simulink model "TotalControllerSimOld"  (R2015b)
settings: Solver=VariableStepAuto  StartTime=0.0  StopTime=t  RelTol=1e-3
values from neighbouring files (symbols this model uses):
  A12 = A(1:3,4:6)    [StateSpace.m]
  Fg = 9.81 * m    (= 9.77076)    [Parameters.m]
  Jx_changed = Jx*5    (= 0.0535)    [Parameters.m]
  Jy_changed = Jy*3    (= 0.0321)    [Parameters.m]
  Jz_changed = Jz*2    (= 0.0427)    [Parameters.m]
  kd = 9.39741e-7    (= 9.39741e-07)    [Parameters.m]
  kth = 1.32922e-5    (= 1.32922e-05)    [Parameters.m]
  L = 0.225    [Parameters.m]
  Lobs = (-place(A22',A12',[-11 -12 -13]))'    [StateSpace.m]
  m = 0.996    [Parameters.m]
  motor_tau = ts/3    (= 0.000333333333333)    [TotalController.m]
  pitch_init = 0    [plotPaper.m]    (also in plotPoster.m; plotStateSpace.m = 0.2; plotTrans.m)
  pitch_ref_time = 0    [plotPaper.m]    (also in plotPoster.m; plotStateSpace.m; plotTrans.m)
  pitch_step = 0    [plotPaper.m]    (also in plotPoster.m; plotStateSpace.m; plotTrans.m)
  roll_init = 0    [plotPaper.m]    (also in plotPoster.m; plotStateSpace.m = -0.3; plotTrans.m)
  roll_ref_time = 0    [plotPaper.m]    (also in plotPoster.m; plotStateSpace.m; plotTrans.m)
  roll_step = 0.2    [plotPaper.m]    (also in plotPoster.m = 0; plotStateSpace.m = 0; plotTrans.m = 0)
  w1_bar = sqrt(Fg/kth/4)    [Parameters.m]
  w2_bar = sqrt(Fg/kth/4)    [Parameters.m]
  w3_bar = sqrt(Fg/kth/4)    [Parameters.m]
  w4_bar = sqrt(Fg/kth/4)    [Parameters.m]
  w_max = 230    [TotalController.m]
  w_min = -161    [TotalController.m]
  x_ref_step = 1    [plotPaper.m]    (also in plotPoster.m = 0; plotStateSpace.m = 0; plotTrans.m)
  x_ref_time = 0    [plotPaper.m]    (also in plotPoster.m; plotStateSpace.m; plotTrans.m)
  xdot_ref_step = 0    [plotPaper.m]    (also in plotPoster.m; plotStateSpace.m; plotTrans.m)
  xdot_ref_time = 0    [plotPaper.m]    (also in plotPoster.m; plotStateSpace.m; plotTrans.m)
  y_ref_step = 1    [plotPaper.m]    (also in plotPoster.m = 0; plotStateSpace.m = 0; plotTrans.m = 0)
  y_ref_time = 8    [plotPaper.m]    (also in plotPoster.m = 0; plotStateSpace.m = 0; plotTrans.m = 2.5)
  yaw_init = 0    [plotPaper.m]    (also in plotPoster.m; plotStateSpace.m = -0.2; plotTrans.m)
  ydot_ref_step = 0    [plotPaper.m]    (also in plotPoster.m; plotStateSpace.m; plotTrans.m)
  ydot_ref_time = 0    [plotPaper.m]    (also in plotPoster.m; plotStateSpace.m; plotTrans.m)
  z_ref_step = 1    [plotPaper.m]    (also in plotPoster.m; plotStateSpace.m = 0; plotTrans.m)
  z_ref_time = 16    [plotPaper.m]    (also in plotPoster.m = 0; plotStateSpace.m = 0; plotTrans.m = 0)
  zdot_ref_step = 0    [plotPaper.m]    (also in plotPoster.m; plotStateSpace.m; plotTrans.m)
  zdot_ref_time = 0    [plotPaper.m]    (also in plotPoster.m; plotStateSpace.m; plotTrans.m)
undefined symbols (not defined in the file or in its folder): ZigBee
libraries: truetime x21, cstblocks x6, simulink x3
settings Model: Creator=USUARIO  LastModifiedBy=USUARIO

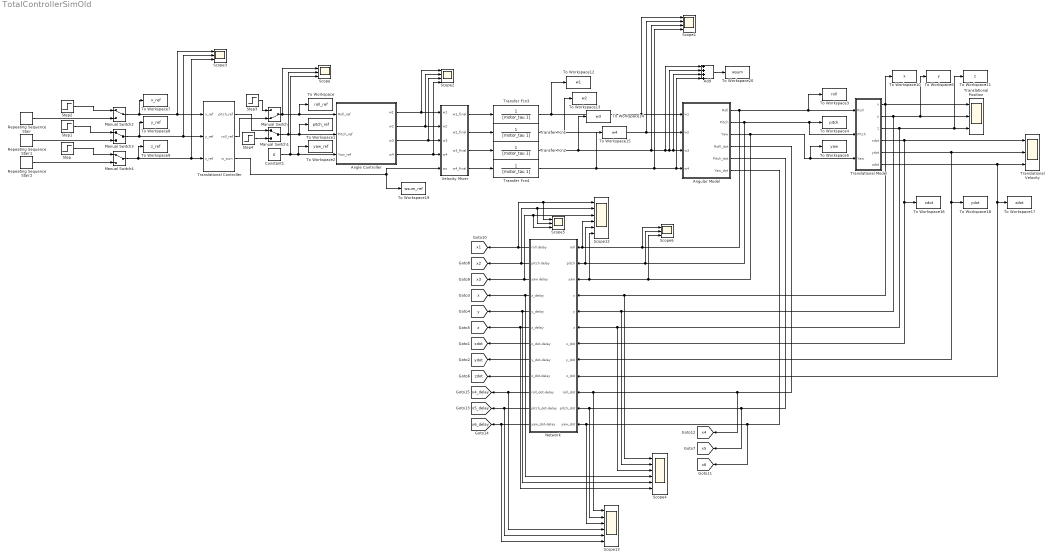
== system TotalControllerSimOld ==
  Add : Sum  Inputs=++++
  Angle Controller : Subsystem
  Angular Model : Subsystem
  Constant1 : Constant  Value=0
  Manual Switch : ManualSwitch  CurrentSetting=0
  Manual Switch{1..4} (4 alike) : ManualSwitch
  Network : Subsystem
  Repeating Sequence Stair : simulink/Sources/Repeating Sequence Stair  OutValues=input_x  tsamp=Tstep  OutMin=[]  OutMax=[]  OutDataTypeStr=double  OutputDataTypeScalingMode=double  OutDataType=fixdt(0,8)  ConRadixGroup=Best Precision: Vector-wise  OutScaling=2^-12
  Repeating Sequence Stair1 : simulink/Sources/Repeating Sequence Stair  OutValues=input_y  tsamp=Tstep  OutMin=[]  OutMax=[]  OutDataTypeStr=double  OutputDataTypeScalingMode=double  OutDataType=fixdt(0,8)  ConRadixGroup=Best Precision: Vector-wise  OutScaling=2^-12
  Repeating Sequence Stair2 : simulink/Sources/Repeating Sequence Stair  OutValues=input_z  tsamp=Tstep  OutMin=[]  OutMax=[]  OutDataTypeStr=double  OutputDataTypeScalingMode=double  OutDataType=fixdt(0,8)  ConRadixGroup=Best Precision: Vector-wise  OutScaling=2^-12
  Scope{,3,5..6} (4 alike) : Scope  NumInputPorts=3
  Scope1 : Scope  NumInputPorts=4
  Scope12 : Scope  NumInputPorts=6
  Scope13 : Scope  NumInputPorts=6
  Scope2 : Scope  NumInputPorts=4
  Scope4 : Scope  NumInputPorts=6
  Step : Step  Time=z_ref_time  After=z_ref_step  SampleTime=0
  Step1 : Step  Time=y_ref_time  After=y_ref_step  SampleTime=0
  Step2 : Step  Time=x_ref_time  After=x_ref_step  SampleTime=0
  Step3 : Step  Time=roll_ref_time  After=roll_step  SampleTime=0
  Step4 : Step  Time=pitch_ref_time  After=pitch_step  SampleTime=0
  To Workspace : ToWorkspace  VariableName=roll_ref  SaveFormat=Timeseries  SampleTime=-1
  To Workspace1 : ToWorkspace  VariableName=pitch_ref  SaveFormat=Timeseries  SampleTime=-1
  To Workspace10 : ToWorkspace  VariableName=x  SaveFormat=Timeseries  SampleTime=-1
  To Workspace11 : ToWorkspace  VariableName=z  SaveFormat=Timeseries  SampleTime=-1
  To Workspace12 : ToWorkspace  VariableName=w1  SaveFormat=Timeseries  SampleTime=-1
  To Workspace13 : ToWorkspace  VariableName=w2  SaveFormat=Timeseries  SampleTime=-1
  To Workspace14 : ToWorkspace  VariableName=w3  SaveFormat=Timeseries  SampleTime=-1
  To Workspace15 : ToWorkspace  VariableName=w4  SaveFormat=Timeseries  SampleTime=-1
  To Workspace16 : ToWorkspace  VariableName=xdot  SaveFormat=Timeseries  SampleTime=-1
  To Workspace17 : ToWorkspace  VariableName=zdot  SaveFormat=Timeseries  SampleTime=-1
  To Workspace18 : ToWorkspace  VariableName=ydot  SaveFormat=Timeseries  SampleTime=-1
  To Workspace19 : ToWorkspace  VariableName=wsum_ref  SaveFormat=Timeseries  SampleTime=-1
  To Workspace2 : ToWorkspace  VariableName=yaw_ref  SaveFormat=Timeseries  SampleTime=-1
  To Workspace20 : ToWorkspace  VariableName=wsum  SaveFormat=Timeseries  SampleTime=-1
  To Workspace3 : ToWorkspace  VariableName=roll  SaveFormat=Timeseries  SampleTime=-1
  To Workspace4 : ToWorkspace  VariableName=pitch  SaveFormat=Timeseries  SampleTime=-1
  To Workspace5 : ToWorkspace  VariableName=yaw  SaveFormat=Timeseries  SampleTime=-1
  To Workspace6 : ToWorkspace  VariableName=y  SaveFormat=Timeseries  SampleTime=-1
  To Workspace7 : ToWorkspace  VariableName=x_ref  SaveFormat=Timeseries  SampleTime=0.035
  To Workspace8 : ToWorkspace  VariableName=y_ref  SaveFormat=Timeseries  SampleTime=0.035
  To Workspace9 : ToWorkspace  VariableName=z_ref  SaveFormat=Timeseries  SampleTime=0.035
  Transfer Fcn{1..4} (4 alike) : TransferFcn  Denominator=[motor_tau 1]
  Translational Controller : Subsystem
  Translational Position : Scope  NumInputPorts=3
  Translational Velocity : Scope  NumInputPorts=3
  Translational Model : Subsystem
  Velocity Mixer : Subsystem
  tag scope: x1=global, x2=global, x3=global, x4=global, x4_delay=global, x5=global, x5_delay=global, x6=global, x6_delay=global, x=global, xdot=global, y=global, ydot=global, z=global, zdot=global
  wires:
  Constant1/1 -> Scope/3, To Workspace2/1, Angle Controller/3(Yaw_ref)
  Velocity Mixer/1(w1_final) -> Transfer Fcn3/1
  Velocity Mixer/2(w2_final) -> Transfer Fcn1/1
  Velocity Mixer/3(w3_final) -> Transfer Fcn2/1
  Velocity Mixer/4(w4_final) -> Transfer Fcn4/1
  Angle Controller/1(w1) -> Velocity Mixer/1(w1), Scope2/1
  Angle Controller/2(w2) -> Velocity Mixer/2(w2), Scope2/2
  Angle Controller/3(w3) -> Scope2/3, Velocity Mixer/3(w3)
  Angle Controller/4(w4) -> Velocity Mixer/4(w4), Scope2/4
  Angular Model/1(Roll) -> Scope12/4, Network/1(roll), Scope6/1, Translational Model/1(Roll), To Workspace3/1
  Angular Model/2(Pitch) -> Scope12/5, Network/2(pitch), Scope6/2, Translational Model/2(Pitch), To Workspace4/1
  Translational Model/1(x) -> Translational Position/1, Network/4(x), Scope4/1, To Workspace10/1
  Translational Model/2(y) -> Translational Position/2, To Workspace6/1, Network/5(y), Scope4/2
  Translational Model/3(z) -> To Workspace11/1, Translational Position/3, Network/6(z), Scope4/3
  Translational Model/4(xdot) -> Network/7(x_dot), To Workspace16/1, Translational Velocity/1
  Translational Model/5(ydot) -> Network/8(y_dot), To Workspace18/1, Translational Velocity/2
  Manual Switch1/1 -> Scope/2, To Workspace1/1, Angle Controller/2(Pitch_ref)
  Network/2(pitch delay) -> Scope5/2, Scope12/2, [x2]
  Network/1(roll delay) -> Scope5/1, Scope12/1, [x1]
  Network/3(yaw delay) -> Scope5/3, Scope12/3, [x3]
  Network/4(x_delay) -> Scope4/4, [x]
  Network/5(y_delay) -> [y], Scope4/5
  Network/6(z_delay) -> [z], Scope4/6
  Network/7(x_dot-delay) -> [xdot]
  Network/8(y_dot-delay) -> [ydot]
  Network/9(z_dot-delay) -> [zdot]
  Angular Model/3(Yaw) -> Scope12/6, Network/3(yaw), Scope6/3, Translational Model/3("Yaw "), To Workspace5/1
  Translational Model/6(zdot) -> Network/9(z_dot), To Workspace17/1, Translational Velocity/3
  Angular Model/4(Rolll_dot) -> Network/10(roll_dot), Scope13/1, [x4]
  Angular Model/6(Yaw_dot) -> [x6], Network/12(yaw_dot), Scope13/3
  Network/10(roll_dot-delay) -> Scope13/4, [x4_delay]
  Network/11(pitch_dot-delay) -> Scope13/5, [x5_delay]
  Network/12(yaw_dot-delay) -> [x6_delay], Scope13/6
  Angular Model/5(Pitch_dot) -> [x5], Network/11(pitch_dot), Scope13/2
  Manual Switch2/1 -> To Workspace7/1, Scope3/1, Translational Controller/1(x_ref)
  Manual Switch4/1 -> To Workspace9/1, Scope3/3, Translational Controller/3(z_ref)
  Manual Switch3/1 -> To Workspace8/1, Scope3/2, Translational Controller/2(y_ref)
  Translational Controller/3(w_sum) -> Velocity Mixer/5(wz), To Workspace19/1
  Step3/1 -> Manual Switch/1
  Step4/1 -> Manual Switch1/2
  Translational Controller/2(roll_ref) -> Manual Switch/2
  Translational Controller/1(pitch_ref) -> Manual Switch1/1
  Transfer Fcn3/1 -> To Workspace12/1, Scope1/1, Angular Model/1(w1)
  Transfer Fcn1/1 -> To Workspace13/1, Scope1/2, Angular Model/2(w2)
  Transfer Fcn4/1 -> To Workspace15/1, Scope1/4, Add/4, Angular Model/4(w4)
  Repeating Sequence Stair/1 -> Manual Switch2/2
  Repeating Sequence Stair1/1 -> Manual Switch3/2
  Repeating Sequence Stair2/1 -> Manual Switch4/2
  Step/1 -> Manual Switch4/1
  Step1/1 -> Manual Switch3/1
  Step2/1 -> Manual Switch2/1
  Manual Switch/1 -> Scope/1, To Workspace/1, Angle Controller/1(Roll_ref)
  Transfer Fcn2/1 -> Scope1/3, Add/1, Add/2, Add/3, Angular Model/3(w3), To Workspace14/1
  Add/1 -> To Workspace20/1

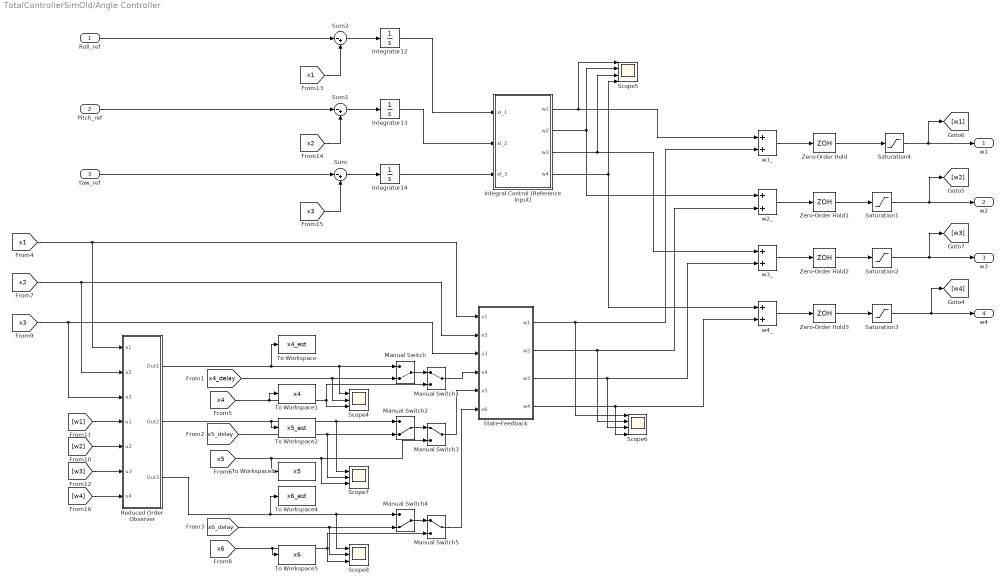
== system TotalControllerSimOld/Angle Controller ==
  Roll_ref : Inport
  Pitch_ref : Inport  Port=2
  Yaw_ref : Inport  Port=3
  Integral Control (Reference Input) : MATLAB Function  TreatAsAtomicUnit=on
  Integrator12 : Integrator
  Integrator13 : Integrator
  Integrator14 : Integrator
  Manual Switch : ManualSwitch  CurrentSetting=0
  Manual Switch1 : ManualSwitch
  Manual Switch2 : ManualSwitch  CurrentSetting=0
  Manual Switch3 : ManualSwitch
  Manual Switch4 : ManualSwitch  CurrentSetting=0
  Manual Switch5 : ManualSwitch
  Reduced Order Observer : Subsystem
  Saturation{1..4} (4 alike) : Saturate  UpperLimit=w_max  LowerLimit=w_min
  Scope4 : Scope  NumInputPorts=3
  Scope5 : Scope  NumInputPorts=4
  Scope6 : Scope  NumInputPorts=4
  Scope7 : Scope  NumInputPorts=3
  Scope8 : Scope  NumInputPorts=3
  "State-Feedback " : MATLAB Function  TreatAsAtomicUnit=on
  Sum : Sum  Inputs=|-+
  Sum1 : Sum  Inputs=|-+
  Sum2 : Sum  Inputs=|-+
  To Workspace : ToWorkspace  VariableName=x4_est  SaveFormat=Timeseries  SampleTime=-1
  To Workspace1 : ToWorkspace  VariableName=x4  SaveFormat=Timeseries  SampleTime=-1
  To Workspace2 : ToWorkspace  VariableName=x5_est  SaveFormat=Timeseries  SampleTime=-1
  To Workspace3 : ToWorkspace  VariableName=x5  SaveFormat=Timeseries  SampleTime=-1
  To Workspace4 : ToWorkspace  VariableName=x6_est  SaveFormat=Timeseries  SampleTime=-1
  To Workspace5 : ToWorkspace  VariableName=x6  SaveFormat=Timeseries  SampleTime=-1
  Zero-Order Hold{,1..3} (4 alike) : ZeroOrderHold  SampleTime=0.035
  w1_ : Sum
  w2_ : Sum
  w3_ : Sum
  w4_ : Sum
  w1 : Outport
  w2 : Outport  Port=2
  w3 : Outport  Port=3
  w4 : Outport  Port=4
  wires:
  "State-Feedback "/4(w4) -> w4_/2, Scope6/4
  Roll_ref/1 -> Sum2/1
  [x3] -> Sum/2
  [x1] -> Sum2/2
  Integrator13/1 -> Integral Control (Reference Input)/2(xI_2)
  "State-Feedback "/1(w1) -> w1_/2, Scope6/1
  [w3] -> Reduced Order Observer/6(u3)
  Sum2/1 -> Integrator12/1
  Sum/1 -> Integrator14/1
  [x3] -> "State-Feedback "/3(x3), Reduced Order Observer/3(x3)
  [w2] -> Reduced Order Observer/5(u2)
  Pitch_ref/1 -> Sum1/1
  Integrator14/1 -> Integral Control (Reference Input)/3(xI_3)
  [x4] -> To Workspace1/1, Scope4/3, Manual Switch1/2
  "State-Feedback "/2(w2) -> w2_/2, Scope6/2
  Integral Control (Reference Input)/2(w2) -> Scope5/2, w2_/1
  [w4] -> Reduced Order Observer/7(u4)
  Integral Control (Reference Input)/3(w3) -> w3_/1, Scope5/3
  [x1] -> "State-Feedback "/1(x1), Reduced Order Observer/1(x1)
  [w1] -> Reduced Order Observer/4(u1)
  Integrator12/1 -> Integral Control (Reference Input)/1(xI_1)
  [x2] -> Sum1/2
  Integral Control (Reference Input)/4(w4) -> Scope5/4, w4_/1
  Integral Control (Reference Input)/1(w1) -> w1_/1, Scope5/1
  [x2] -> "State-Feedback "/2(x2), Reduced Order Observer/2(x2)
  Sum1/1 -> Integrator13/1
  Yaw_ref/1 -> Sum/1
  "State-Feedback "/3(w3) -> w3_/2, Scope6/3
  w1_/1 -> Zero-Order Hold/1
  w4_/1 -> Zero-Order Hold3/1
  w2_/1 -> Zero-Order Hold1/1
  w3_/1 -> Zero-Order Hold2/1
  Zero-Order Hold/1 -> Saturation4/1
  Zero-Order Hold1/1 -> Saturation1/1
  Zero-Order Hold2/1 -> Saturation2/1
  Zero-Order Hold3/1 -> Saturation3/1
  Saturation4/1 -> w1/1, [w1]
  Saturation1/1 -> w2/1, [w2]
  Saturation2/1 -> w3/1, [w3]
  Saturation3/1 -> w4/1, [w4]
  Manual Switch/1 -> Manual Switch1/1
  Manual Switch2/1 -> Manual Switch3/1
  Manual Switch4/1 -> Manual Switch5/1
  Manual Switch1/1 -> "State-Feedback "/4(x4)
  Manual Switch3/1 -> "State-Feedback "/5(x5)
  Manual Switch5/1 -> "State-Feedback "/6(x6)
  Reduced Order Observer/1(Out1) -> To Workspace/1, Scope4/1, Manual Switch/1
  Reduced Order Observer/2(Out2) -> To Workspace2/1, Scope7/1, Manual Switch2/1
  Reduced Order Observer/3(Out3) -> To Workspace4/1, Scope8/1, Manual Switch4/1
  [x4_delay] -> Scope4/2, Manual Switch/2
  [x5_delay] -> Scope7/2, Manual Switch2/2
  [x6_delay] -> Scope8/2, Manual Switch4/2
  [x6] -> To Workspace5/1, Manual Switch5/2, Scope8/3
  [x5] -> To Workspace3/1, Scope7/3, Manual Switch3/2

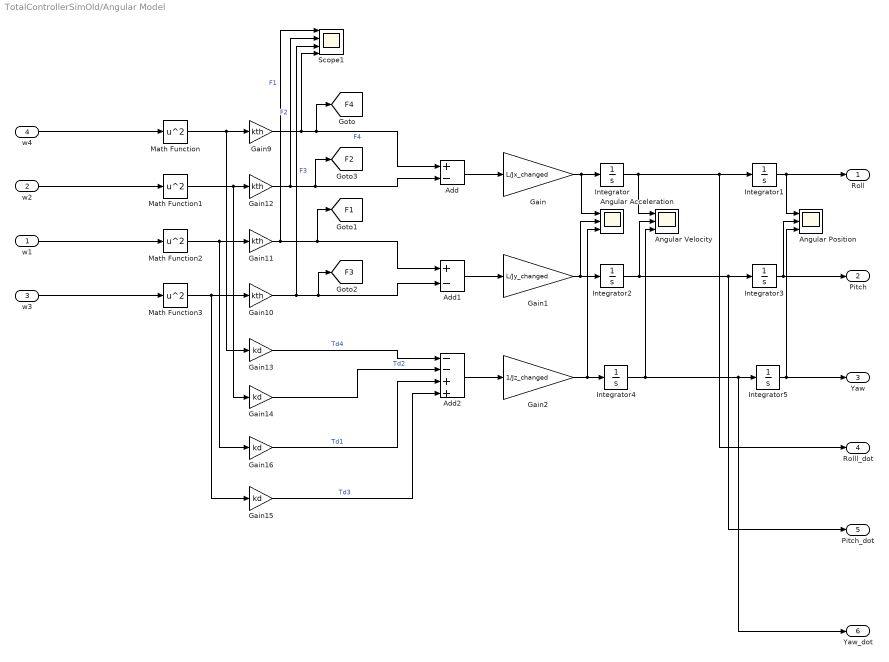
== system TotalControllerSimOld/Angular Model ==
  w1 : Inport
  w2 : Inport  Port=2
  w3 : Inport  Port=3
  w4 : Inport  Port=4
  Add : Sum  Inputs=+-
  Add1 : Sum  Inputs=+-
  Add2 : Sum  Inputs=--++
  Angular Position : Scope  NumInputPorts=3
  Angular Velocity : Scope  NumInputPorts=3
  Angular Acceleration : Scope  NumInputPorts=3
  Gain : Gain  Gain=L/Jx_changed
  Gain1 : Gain  Gain=L/Jy_changed
  Gain{9..12} (4 alike) : Gain  Gain=kth
  Gain{13..16} (4 alike) : Gain  Gain=kd
  Gain2 : Gain  Gain=1/Jz_changed
  Integrator : Integrator
  Integrator1 : Integrator  InitialCondition=roll_init
  Integrator2 : Integrator
  Integrator3 : Integrator  InitialCondition=pitch_init
  Integrator4 : Integrator
  Integrator5 : Integrator  InitialCondition=yaw_init
  Math Function{,1..3} (4 alike) : Math  Operator=square  SaturateOnIntegerOverflow=on
  Scope1 : Scope  NumInputPorts=4
  Roll : Outport
  Pitch : Outport  Port=2
  Yaw : Outport  Port=3
  Rolll_dot : Outport  Port=4
  Pitch_dot : Outport  Port=5
  Yaw_dot : Outport  Port=6
  tag scope: F1=global, F2=global, F3=global, F4=global
  wires:
  Gain1/1 -> Angular Acceleration/2, Integrator2/1
  Add2/1 -> Gain2/1
  Gain9/1 -> Scope1/4, [F4], Add/1  "F4"
  Gain14/1 -> Add2/2  "Td2"
  Gain16/1 -> Add2/3  "Td1"
  Gain/1 -> Angular Acceleration/1, Integrator/1
  Integrator/1 -> Angular Velocity/1, Rolll_dot/1, Integrator1/1
  Integrator1/1 -> Roll/1, Angular Position/1
  Integrator4/1 -> Angular Velocity/3, Yaw_dot/1, Integrator5/1
  Add/1 -> Gain/1
  Integrator3/1 -> Pitch/1, Angular Position/2
  Add1/1 -> Gain1/1
  Integrator5/1 -> Angular Position/3, Yaw/1
  Gain12/1 -> Scope1/2, [F2], Add/2  "F2"
  Gain10/1 -> [F3], Add1/2, Scope1/3  "F3"
  Gain11/1 -> Scope1/1, [F1], Add1/1  "F1"
  Gain13/1 -> Add2/1  "Td4"
  Gain15/1 -> Add2/4  "Td3"
  Integrator2/1 -> Angular Velocity/2, Pitch_dot/1, Integrator3/1
  Gain2/1 -> Angular Acceleration/3, Integrator4/1
  Math Function3/1 -> Gain15/1, Gain10/1
  Math Function2/1 -> Gain16/1, Gain11/1
  Math Function/1 -> Gain13/1, Gain9/1
  Math Function1/1 -> Gain14/1, Gain12/1
  w1/1 -> Math Function2/1
  w2/1 -> Math Function1/1
  w3/1 -> Math Function3/1
  w4/1 -> Math Function/1

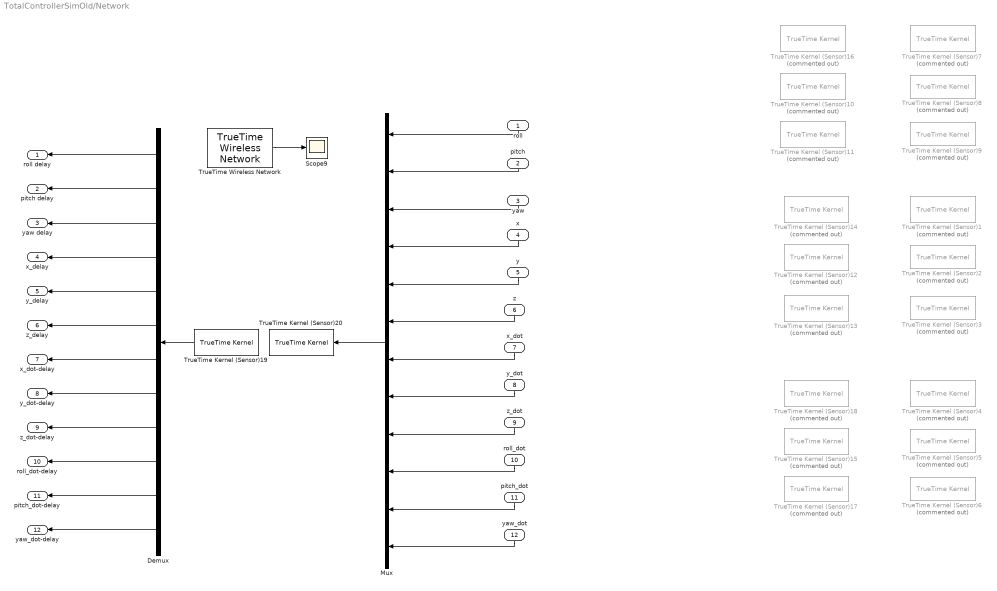
== system TotalControllerSimOld/Network ==
  roll : Inport
  pitch : Inport  Port=2
  yaw : Inport  Port=3
  x : Inport  Port=4
  y : Inport  Port=5
  z : Inport  Port=6
  x_dot : Inport  Port=7
  y_dot : Inport  Port=8
  z_dot : Inport  Port=9
  roll_dot : Inport  Port=10
  pitch_dot : Inport  Port=11
  yaw_dot : Inport  Port=12
  Demux : Demux  Outputs=12
  Mux : Mux  Inputs=12
  Scope9 : Scope
  TrueTime Kernel (Sensor)1 : truetime/TrueTime Kernel  Priority=1  Commented=on  sfun=sensor_init  args=[]  ninputsoutputs=[1 0]  ntriggers=0  trigtype=rising  nwnodenbr=[1 1]  clockoffsetdrift=[0 0]  schedoutput=off  battery=off  poweroutput=off  label=1: 1
  TrueTime Kernel (Sensor)10 : truetime/TrueTime Kernel  Priority=1  Commented=on  sfun=drone_init  args=[]  ninputsoutputs=[0 1]  ntriggers=0  trigtype=rising  nwnodenbr=[1 11]  clockoffsetdrift=[0 0]  schedoutput=off  battery=off  poweroutput=off  label=1: 11
  TrueTime Kernel (Sensor)11 : truetime/TrueTime Kernel  Priority=1  Commented=on  sfun=drone_init  args=[]  ninputsoutputs=[0 1]  ntriggers=0  trigtype=rising  nwnodenbr=[1 12]  clockoffsetdrift=[0 0]  schedoutput=off  battery=off  poweroutput=off  label=1: 12
  TrueTime Kernel (Sensor)12 : truetime/TrueTime Kernel  Priority=1  Commented=on  sfun=drone_init  args=[]  ninputsoutputs=[0 1]  ntriggers=0  trigtype=rising  nwnodenbr=[1 14]  clockoffsetdrift=[0 0]  schedoutput=off  battery=off  poweroutput=off  label=1: 14
  TrueTime Kernel (Sensor)13 : truetime/TrueTime Kernel  Priority=1  Commented=on  sfun=drone_init  args=[]  ninputsoutputs=[0 1]  ntriggers=0  trigtype=rising  nwnodenbr=[1 15]  clockoffsetdrift=[0 0]  schedoutput=off  battery=off  poweroutput=off  label=1: 15
  TrueTime Kernel (Sensor)14 : truetime/TrueTime Kernel  Priority=1  Commented=on  sfun=drone_init  args=[]  ninputsoutputs=[0 1]  ntriggers=0  trigtype=rising  nwnodenbr=[1 13]  clockoffsetdrift=[0 0]  schedoutput=off  battery=off  poweroutput=off  label=1: 13
  TrueTime Kernel (Sensor)15 : truetime/TrueTime Kernel  Priority=1  Commented=on  sfun=drone_init  args=[]  ninputsoutputs=[0 1]  ntriggers=0  trigtype=rising  nwnodenbr=[1 17]  clockoffsetdrift=[0 0]  schedoutput=off  battery=off  poweroutput=off  label=1: 17
  TrueTime Kernel (Sensor)16 : truetime/TrueTime Kernel  Priority=1  Commented=on  sfun=drone_init  args=[]  ninputsoutputs=[0 1]  ntriggers=0  trigtype=rising  nwnodenbr=[1 10]  clockoffsetdrift=[0 0]  schedoutput=off  battery=off  poweroutput=off  label=1: 10
  TrueTime Kernel (Sensor)17 : truetime/TrueTime Kernel  Priority=1  Commented=on  sfun=drone_init  args=[]  ninputsoutputs=[0 1]  ntriggers=0  trigtype=rising  nwnodenbr=[1 18]  clockoffsetdrift=[0 0]  schedoutput=off  battery=off  poweroutput=off  label=1: 18
  TrueTime Kernel (Sensor)18 : truetime/TrueTime Kernel  Priority=1  Commented=on  sfun=drone_init  args=[]  ninputsoutputs=[0 1]  ntriggers=0  trigtype=rising  nwnodenbr=[1 16]  clockoffsetdrift=[0 0]  schedoutput=off  battery=off  poweroutput=off  label=1: 16
  TrueTime Kernel (Sensor)19 : truetime/TrueTime Kernel  Priority=1  sfun=drone_init  args=[]  ninputsoutputs=[0 12]  ntriggers=0  trigtype=rising  nwnodenbr=[1 2]  clockoffsetdrift=[0 0]  schedoutput=off  battery=off  poweroutput=off  label=1: 2
  TrueTime Kernel (Sensor)2 : truetime/TrueTime Kernel  Priority=1  Commented=on  sfun=sensor_init  args=[]  ninputsoutputs=[1 0]  ntriggers=0  trigtype=rising  nwnodenbr=[1 2]  clockoffsetdrift=[0 0]  schedoutput=off  battery=off  poweroutput=off  label=1: 2
  TrueTime Kernel (Sensor)20 : truetime/TrueTime Kernel  Priority=1  sfun=sensor_init  args=[]  ninputsoutputs=[12 0]  ntriggers=0  trigtype=rising  nwnodenbr=[1 1]  clockoffsetdrift=[0 0]  schedoutput=off  battery=off  poweroutput=off  label=1: 1
  TrueTime Kernel (Sensor)3 : truetime/TrueTime Kernel  Priority=1  Commented=on  sfun=sensor_init  args=[]  ninputsoutputs=[1 0]  ntriggers=0  trigtype=rising  nwnodenbr=[1 3]  clockoffsetdrift=[0 0]  schedoutput=off  battery=off  poweroutput=off  label=1: 3
  TrueTime Kernel (Sensor)4 : truetime/TrueTime Kernel  Priority=1  Commented=on  sfun=sensor_init  args=[]  ninputsoutputs=[1 0]  ntriggers=0  trigtype=rising  nwnodenbr=[1 4]  clockoffsetdrift=[0 0]  schedoutput=off  battery=off  poweroutput=off  label=1: 4
  TrueTime Kernel (Sensor)5 : truetime/TrueTime Kernel  Priority=1  Commented=on  sfun=sensor_init  args=[]  ninputsoutputs=[1 0]  ntriggers=0  trigtype=rising  nwnodenbr=[1 5]  clockoffsetdrift=[0 0]  schedoutput=off  battery=off  poweroutput=off  label=1: 5
  TrueTime Kernel (Sensor)6 : truetime/TrueTime Kernel  Priority=1  Commented=on  sfun=sensor_init  args=[]  ninputsoutputs=[1 0]  ntriggers=0  trigtype=rising  nwnodenbr=[1 6]  clockoffsetdrift=[0 0]  schedoutput=off  battery=off  poweroutput=off  label=1: 6
  TrueTime Kernel (Sensor)7 : truetime/TrueTime Kernel  Priority=1  Commented=on  sfun=sensor_init  args=[]  ninputsoutputs=[1 0]  ntriggers=0  trigtype=rising  nwnodenbr=[1 7]  clockoffsetdrift=[0 0]  schedoutput=off  battery=off  poweroutput=off  label=1: 7
  TrueTime Kernel (Sensor)8 : truetime/TrueTime Kernel  Priority=1  Commented=on  sfun=sensor_init  args=[]  ninputsoutputs=[1 0]  ntriggers=0  trigtype=rising  nwnodenbr=[1 8]  clockoffsetdrift=[0 0]  schedoutput=off  battery=off  poweroutput=off  label=1: 8
  TrueTime Kernel (Sensor)9 : truetime/TrueTime Kernel  Priority=1  Commented=on  sfun=sensor_init  args=[]  ninputsoutputs=[1 0]  ntriggers=0  trigtype=rising  nwnodenbr=[1 9]  clockoffsetdrift=[0 0]  schedoutput=off  battery=off  poweroutput=off  label=1: 9
  TrueTime Wireless Network : truetime/TrueTime Wireless  Network  nwtype=802.15.4 (ZigBee)  nwnbr=1  nnodes=2  rate=1000000  minsize=272  transpower=20  threshold=-48  use_pathloss_function=default  pathloss=3.5  acktimeout=0.00004  retrylimit=5  error_threshold=0.03  lossprob=0  seed=0  scheduleoutput=on  poweroutput=off
  roll delay : Outport
  pitch delay : Outport  Port=2
  yaw delay : Outport  Port=3
  x_delay : Outport  Port=4
  y_delay : Outport  Port=5
  z_delay : Outport  Port=6
  x_dot-delay : Outport  Port=7
  y_dot-delay : Outport  Port=8
  z_dot-delay : Outport  Port=9
  roll_dot-delay : Outport  Port=10
  pitch_dot-delay : Outport  Port=11
  yaw_dot-delay : Outport  Port=12
  wires:
  TrueTime Wireless Network/1 -> Scope9/1
  Demux/1 -> roll delay/1
  Demux/2 -> pitch delay/1
  Demux/3 -> yaw delay/1
  Demux/4 -> x_delay/1
  Demux/5 -> y_delay/1
  Demux/6 -> z_delay/1
  Demux/7 -> x_dot-delay/1
  Demux/8 -> y_dot-delay/1
  Demux/9 -> z_dot-delay/1
  x_dot/1 -> Mux/7
  y_dot/1 -> Mux/8
  z/1 -> Mux/6
  y/1 -> Mux/5
  x/1 -> Mux/4
  yaw/1 -> Mux/3
  pitch/1 -> Mux/2
  roll/1 -> Mux/1
  Mux/1 -> TrueTime Kernel (Sensor)20/1
  TrueTime Kernel (Sensor)19/1 -> Demux/1
  Demux/10 -> roll_dot-delay/1
  Demux/11 -> pitch_dot-delay/1
  Demux/12 -> yaw_dot-delay/1
  roll_dot/1 -> Mux/10
  yaw_dot/1 -> Mux/12
  pitch_dot/1 -> Mux/11
  z_dot/1 -> Mux/9

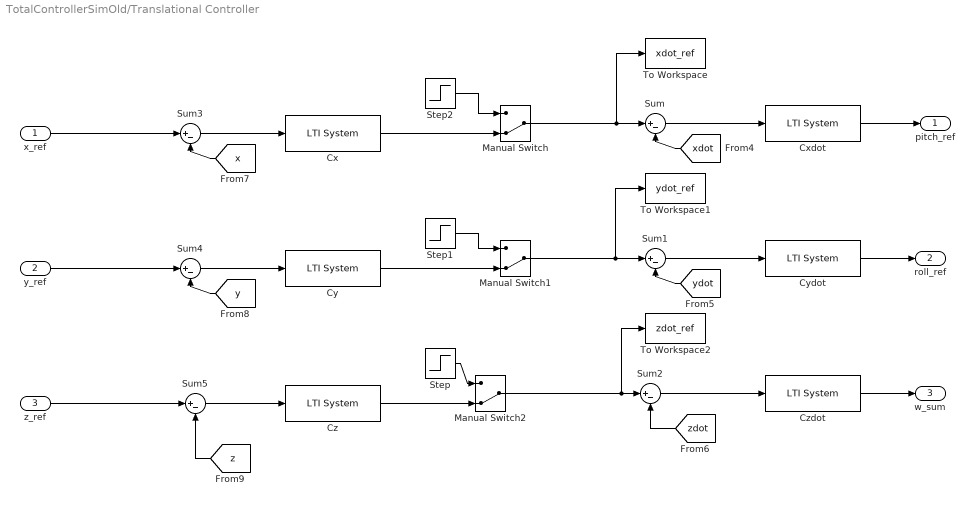
== system TotalControllerSimOld/Translational Controller ==
  x_ref : Inport
  y_ref : Inport  Port=2
  z_ref : Inport  Port=3
  Cx : cstblocks/LTI System  sys=Cx  IC=[]
  Cxdot : cstblocks/LTI System  sys=Cxdot  IC=[]
  Cy : cstblocks/LTI System  sys=Cy  IC=[]
  Cydot : cstblocks/LTI System  sys=Cydot  IC=[]
  "Cz " : cstblocks/LTI System  sys=Cz  IC=[]
  Czdot : cstblocks/LTI System  sys=Czdot  IC=[]
  Manual Switch : ManualSwitch  CurrentSetting=0
  Manual Switch1 : ManualSwitch  CurrentSetting=0
  Manual Switch2 : ManualSwitch  CurrentSetting=0
  Step : Step  Time=zdot_ref_time  After=zdot_ref_step  SampleTime=0
  Step1 : Step  Time=ydot_ref_time  After=ydot_ref_step  SampleTime=0
  Step2 : Step  Time=xdot_ref_time  After=xdot_ref_step  SampleTime=0
  Sum{,1..5} (6 alike) : Sum  Inputs=|+-
  To Workspace : ToWorkspace  VariableName=xdot_ref  SaveFormat=Timeseries  SampleTime=-1
  To Workspace1 : ToWorkspace  VariableName=ydot_ref  SaveFormat=Timeseries  SampleTime=-1
  To Workspace2 : ToWorkspace  VariableName=zdot_ref  SaveFormat=Timeseries  SampleTime=-1
  pitch_ref : Outport
  roll_ref : Outport  Port=2
  w_sum : Outport  Port=3
  wires:
  Cxdot/1 -> pitch_ref/1
  Cydot/1 -> roll_ref/1
  Sum/1 -> Cxdot/1
  Sum4/1 -> Cy/1
  Sum1/1 -> Cydot/1
  Manual Switch2/1 -> To Workspace2/1, Sum2/1
  Sum3/1 -> Cx/1
  [ydot] -> Sum1/2
  [y] -> Sum4/2
  Czdot/1 -> w_sum/1
  [x] -> Sum3/2
  x_ref/1 -> Sum3/1
  [xdot] -> Sum/2
  Manual Switch1/1 -> To Workspace1/1, Sum1/1
  z_ref/1 -> Sum5/1
  Manual Switch/1 -> To Workspace/1, Sum/1
  [zdot] -> Sum2/2
  Sum2/1 -> Czdot/1
  Sum5/1 -> "Cz "/1
  [z] -> Sum5/2
  y_ref/1 -> Sum4/1
  Cx/1 -> Manual Switch/2
  Cy/1 -> Manual Switch1/2
  "Cz "/1 -> Manual Switch2/2
  Step2/1 -> Manual Switch/1
  Step1/1 -> Manual Switch1/1
  Step/1 -> Manual Switch2/1

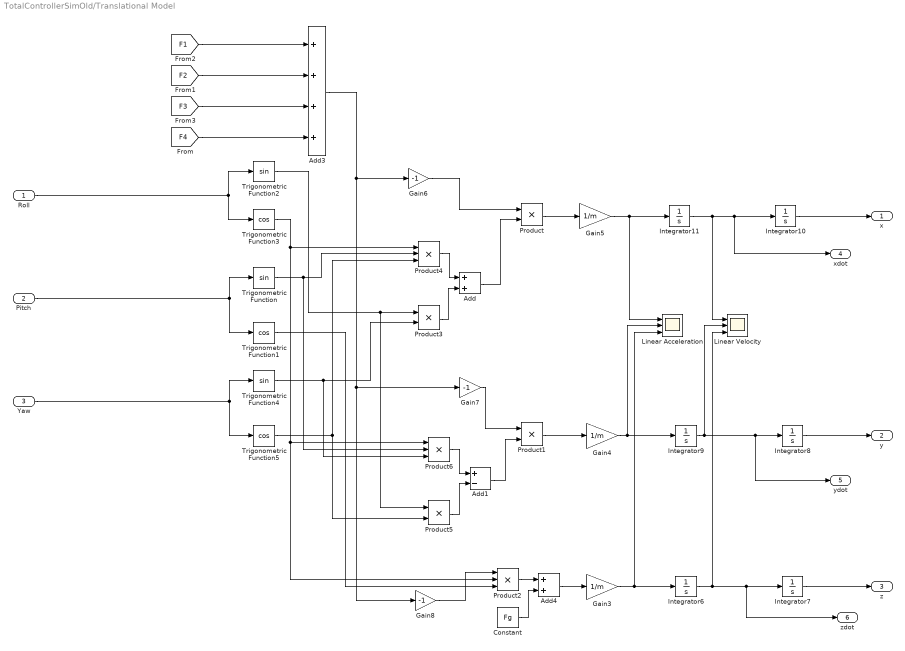
== system TotalControllerSimOld/Translational Model ==
  Roll : Inport
  Pitch : Inport  Port=2
  "Yaw " : Inport  Port=3
  Add : Sum
  Add1 : Sum  Inputs=+-
  Add3 : Sum  Inputs=4
  Add4 : Sum  Inputs=2
  Constant : Constant  Value=Fg
  Gain3 : Gain  Gain=1/m
  Gain4 : Gain  Gain=1/m
  Gain5 : Gain  Gain=1/m
  Gain6 : Gain  Gain=-1
  Gain7 : Gain  Gain=-1
  Gain8 : Gain  Gain=-1
  Integrator{6..11} (6 alike) : Integrator
  Linear Acceleration : Scope  NumInputPorts=3
  Linear Velocity : Scope  NumInputPorts=3
  Product{,1,3,5} (4 alike) : Product
  Product2 : Product  Inputs=3
  Product4 : Product  Inputs=3
  Product6 : Product  Inputs=3
  Trigonometric Function : Trigonometry
  Trigonometric Function1 : Trigonometry  Operator=cos
  Trigonometric Function2 : Trigonometry
  Trigonometric Function3 : Trigonometry  Operator=cos
  Trigonometric Function4 : Trigonometry
  Trigonometric Function5 : Trigonometry  Operator=cos
  x : Outport
  y : Outport  Port=2
  z : Outport  Port=3
  xdot : Outport  Port=4
  ydot : Outport  Port=5
  zdot : Outport  Port=6
  wires:
  Integrator11/1 -> xdot/1, Integrator10/1, Linear Velocity/1
  Integrator7/1 -> z/1
  Gain5/1 -> Integrator11/1, Linear Acceleration/1
  Integrator9/1 -> ydot/1, Integrator8/1, Linear Velocity/2
  Integrator10/1 -> x/1
  Integrator8/1 -> y/1
  [F3] -> Add3/3
  Product/1 -> Gain5/1
  Product1/1 -> Gain4/1
  Gain4/1 -> Integrator9/1, Linear Acceleration/2
  Integrator6/1 -> zdot/1, Integrator7/1, Linear Velocity/3
  Gain7/1 -> Product1/1
  Trigonometric Function2/1 -> Product5/1, Product3/1
  Constant/1 -> Add4/2
  [F4] -> Add3/4
  Add3/1 -> Gain8/1, Gain7/1, Gain6/1
  [F2] -> Add3/2
  Trigonometric Function1/1 -> Product2/3
  [F1] -> Add3/1
  Product2/1 -> Add4/1
  Add4/1 -> Gain3/1
  Gain6/1 -> Product/1
  Gain8/1 -> Product2/1
  Trigonometric Function3/1 -> Product4/1, Product6/1, Product2/2
  Gain3/1 -> Integrator6/1, Linear Acceleration/3
  Roll/1 -> Trigonometric Function3/1, Trigonometric Function2/1
  Pitch/1 -> Trigonometric Function/1, Trigonometric Function1/1
  Add/1 -> Product/2
  Product3/1 -> Add/2
  Product4/1 -> Add/1
  "Yaw "/1 -> Trigonometric Function4/1, Trigonometric Function5/1
  Trigonometric Function/1 -> Product6/2, Product4/2
  Trigonometric Function5/1 -> Product4/3, Product5/2
  Trigonometric Function4/1 -> Product6/3, Product3/2
  Product5/1 -> Add1/2
  Product6/1 -> Add1/1
  Add1/1 -> Product1/2

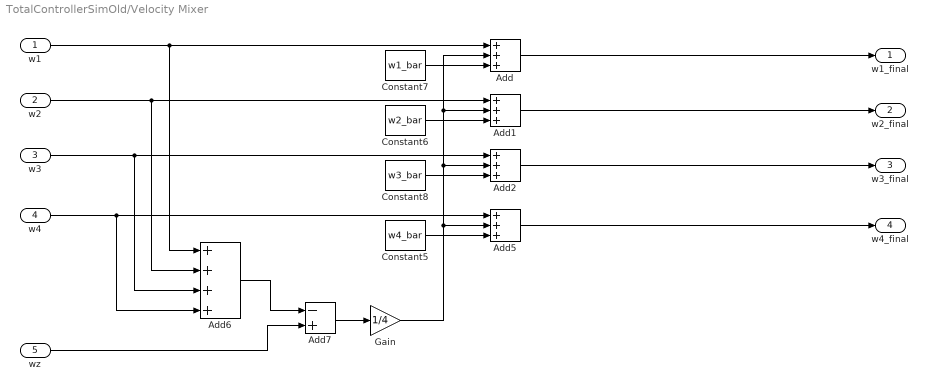
== system TotalControllerSimOld/Velocity Mixer ==
  w1 : Inport
  w2 : Inport  Port=2
  w3 : Inport  Port=3
  w4 : Inport  Port=4
  wz : Inport  Port=5
  Add{,1..2,5} (4 alike) : Sum  Inputs=+++
  Add6 : Sum  Inputs=4
  Add7 : Sum  Inputs=-+
  Constant5 : Constant  Value=w4_bar
  Constant6 : Constant  Value=w2_bar
  Constant7 : Constant  Value=w1_bar
  Constant8 : Constant  Value=w3_bar
  Gain : Gain  Gain=1/4
  w1_final : Outport
  w2_final : Outport  Port=2
  w3_final : Outport  Port=3
  w4_final : Outport  Port=4
  wires:
  w4/1 -> Add6/4, Add5/1
  Gain/1 -> Add5/2, Add2/2, Add/2, Add1/2
  Add7/1 -> Gain/1
  Add6/1 -> Add7/1
  w2/1 -> Add6/2, Add1/1
  w3/1 -> Add6/3, Add2/1
  wz/1 -> Add7/2
  w1/1 -> Add/1, Add6/1
  Constant7/1 -> Add/3
  Constant6/1 -> Add1/3
  Constant8/1 -> Add2/3
  Constant5/1 -> Add5/3
  Add/1 -> w1_final/1
  Add1/1 -> w2_final/1
  Add2/1 -> w3_final/1
  Add5/1 -> w4_final/1

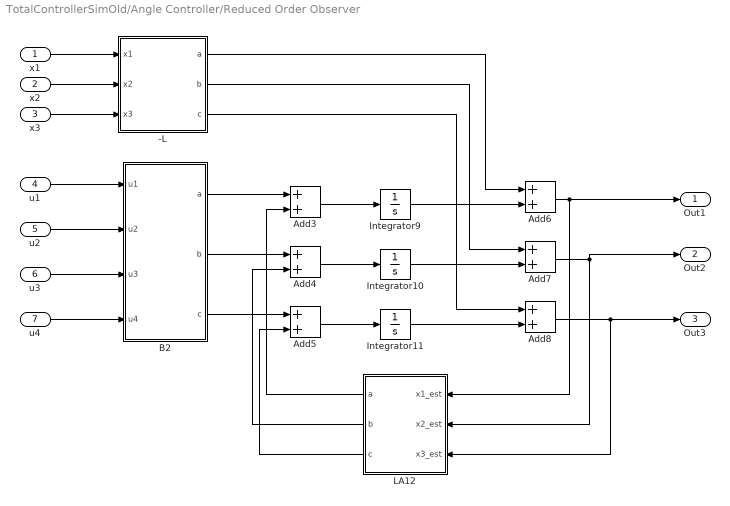
== system TotalControllerSimOld/Angle Controller/Reduced Order Observer ==
  x1 : Inport
  x2 : Inport  Port=2
  x3 : Inport  Port=3
  u1 : Inport  Port=4
  u2 : Inport  Port=5
  u3 : Inport  Port=6
  u4 : Inport  Port=7
  "-L " : MATLAB Function  TreatAsAtomicUnit=on
  Add{3..8} (6 alike) : Sum  Inputs=2
  B2 : MATLAB Function  TreatAsAtomicUnit=on
  Integrator10 : Integrator
  Integrator11 : Integrator
  Integrator9 : Integrator
  LA12 : MATLAB Function  TreatAsAtomicUnit=on
  Out1 : Outport
  Out2 : Outport  Port=2
  Out3 : Outport  Port=3
  wires:
  Add4/1 -> Integrator10/1
  Add3/1 -> Integrator9/1
  Add5/1 -> Integrator11/1
  u4/1 -> B2/4(u4)
  u2/1 -> B2/2(u2)
  B2/1(a) -> Add3/1
  B2/2(b) -> Add4/1
  B2/3(c) -> Add5/1
  LA12/1(a) -> Add3/2
  LA12/2(b) -> Add4/2
  LA12/3(c) -> Add5/2
  Add6/1 -> LA12/1(x1_est), Out1/1
  Add7/1 -> LA12/2(x2_est), Out2/1
  Add8/1 -> LA12/3(x3_est), Out3/1
  "-L "/3(c) -> Add8/1
  "-L "/1(a) -> Add6/1
  "-L "/2(b) -> Add7/1
  x2/1 -> "-L "/2(x2)
  x3/1 -> "-L "/3(x3)
  x1/1 -> "-L "/1(x1)
  Integrator9/1 -> Add6/2
  Integrator11/1 -> Add8/2
  Integrator10/1 -> Add7/2
  u1/1 -> B2/1(u1)
  u3/1 -> B2/3(u3)

== matlab function TotalControllerSimOld/Angle Controller/State-Feedback  ==
  data: x1 input; w1 output; w2 output; w3 output; w4 output; x2 input; x3 input; x4 input; x5 input; x6 input; F parameter
function [w1,w2,w3,w4] = F_matrix(x1, x2, x3, x4, x5, x6, F)
x=[x1;
    x2;
    x3;
    x4;
    x5;
    x6];

w=F*x;

w1=w(1);
w2=w(2);
w3=w(3);
w4=w(4);

== matlab function TotalControllerSimOld/Angle Controller/Integral Control (Reference Input) ==
  data: xI_1 input; w1 output; w2 output; w3 output; w4 output; xI_2 input; xI_3 input; FI parameter
function [w1,w2,w3,w4] = FI_matrix(xI_1, xI_2, xI_3,FI)
xI=[xI_1;
    xI_2;
    xI_3];

w=FI*xI;

w1=w(1);
w2=w(2);
w3=w(3);
w4=w(4);

== matlab function TotalControllerSimOld/Angle Controller/Reduced Order Observer/-L  ==
  data: x1 input; a output; b output; c output; x2 input; x3 input; Lobs parameter
function [a,b,c] = minusL_matrix(x1, x2, x3, Lobs)
x=[x1;
    x2;
    x3];

abc=-Lobs*x;

a=abc(1);
b=abc(2);
c=abc(3);

== matlab function TotalControllerSimOld/Angle Controller/Reduced Order Observer/B2 ==
  data: u1 input; a output; b output; c output; u2 input; u3 input; u4 input; B2 parameter
function [a, b, c] = B2_matrix(u1, u2, u3, u4, B2)
u=[u1;
    u2;
    u3;
    u4];

abc=B2*u;

a=abc(1);
b=abc(2);
c=abc(3);

== matlab function TotalControllerSimOld/Angle Controller/Reduced Order Observer/LA12 ==
  data: x1_est input; x2_est input; x3_est input; a output; b output; c output; Lobs parameter; A12 parameter
function [a,b,c] = LA12_matrix(x1_est, x2_est, x3_est, Lobs, A12)
x=[x1_est;
    x2_est;
    x3_est];

abc=Lobs*A12*x;

a=abc(1);
b=abc(2);
c=abc(3);
